simulink model "hw3_statecharte"  (R2013a)
settings: Solver=ode3  StartTime=0.0  StopTime=10.0  FixedStep=.1  RelTol=1e-3
libraries: simulink x1
settings Model: Creator=eiseles  LastModifiedBy=eiseles

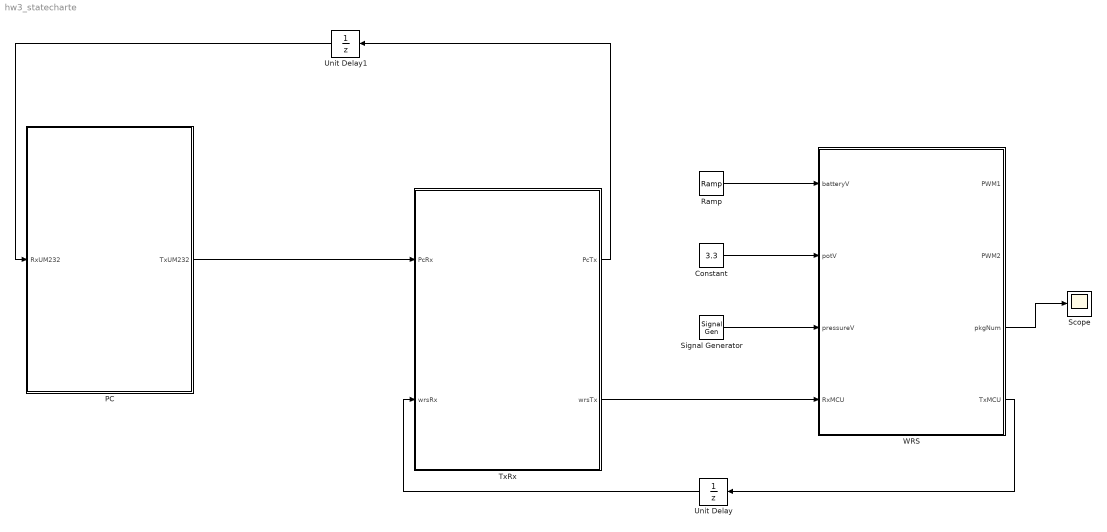
== system hw3_statecharte ==
  Constant : Constant  Value=3.3
  PC : Stateflow chart  TreatAsAtomicUnit=on
  Ramp : simulink/Sources/Ramp  slope=-.1  start=0  X0=5
  Scope : Scope
  Signal Generator : SignalGenerator
  TxRx : Stateflow chart  TreatAsAtomicUnit=on
  Unit Delay : UnitDelay  SampleTime=-1
  Unit Delay1 : UnitDelay  SampleTime=-1
  WRS : Stateflow chart  TreatAsAtomicUnit=on
  wires:
  PC/1(TxUM232) -> TxRx/1(PcRx)
  TxRx/2(wrsTx) -> WRS/4(RxMCU)
  TxRx/1(PcTx) -> Unit Delay1/1
  WRS/4(TxMCU) -> Unit Delay/1
  Unit Delay/1 -> TxRx/2(wrsRx)
  Unit Delay1/1 -> PC/1(RxUM232)
  WRS/3(pkgNum) -> Scope/1
  Ramp/1 -> WRS/1(batteryV)
  Constant/1 -> WRS/2(potV)
  Signal Generator/1 -> WRS/3(pressureV)

== stateflow chart hw3_statecharte/WRS ==
  state Collect [parallel]
    settings: executionOrder=1
    state collectAnalog
      en:pkgNum++;
    (default) -> collectAnalog
    (junction 31) -> collectAnalog [order 1] : [pkgNum%%5==0]
    (junction 31) -> collectAnalog [order 2]
    collectAnalog -> (junction 31) : after(.2,sec)
  data: PWM1 output double; PWM2 output double; pkgNum output double =0; batteryV input; potV input; pressureV input; RxMCU input; TxMCU output

== stateflow chart hw3_statecharte/PC ==
  data: TxUM232 output double; RxUM232 input double

== stateflow chart hw3_statecharte/TxRx ==
  data: PcRx input; PcTx output; wrsRx input; wrsTx output
